simulink model "acc_decision_matlab_function"  (R2024b)
settings: Solver=FixedStepDiscrete  StartTime=0.0  StopTime=0.2  FixedStep=0.05  RelTol=1e-3
settings Model: Creator=aiden  LastModifiedBy=aiden
settings DataIOCC: ExternalInput=command_input, ego_speed_kmh, has_target, current_distance, reset_signal  LoadExternalInput=on

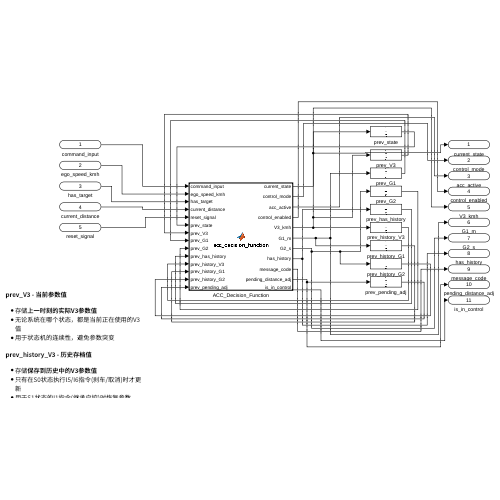
[thumbnail: Simulink's stored preview of the top-level diagram]
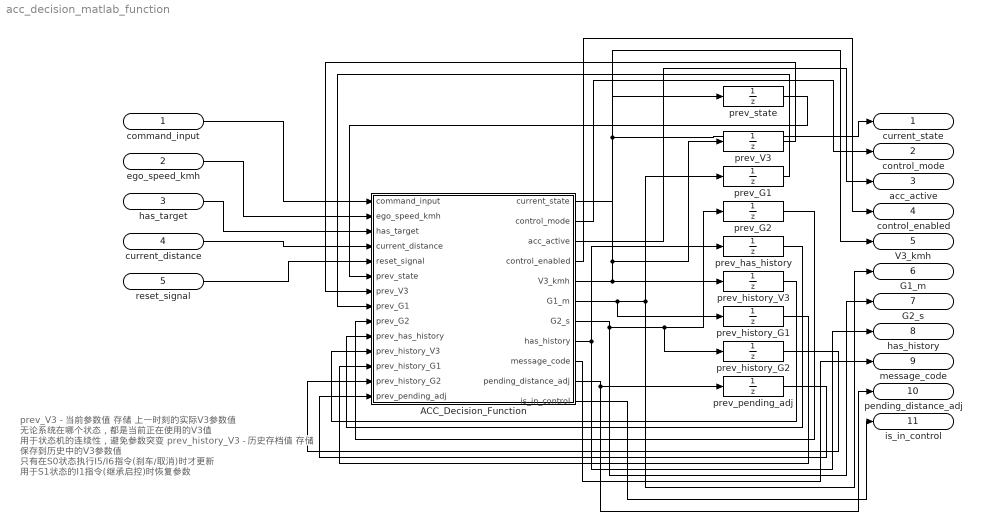
== system acc_decision_matlab_function ==
  note: prev_V3 - 当前参数值
      | 存储 上一时刻的实际V3参数值
      | 无论系统在哪个状态，都是当前正在使用的V3值
      | 用于状态机的连续性，避免参数突变
      | prev_history_V3 - 历史存档值
      | 存储 保存到历史中的V3参数值
      | 只有在S0状态执行I5/I6指令(刹车/取消)时才更新
      | 用于S1状态的I1指令(继承启控)时恢复参数
  command_input : Inport
  ego_speed_kmh : Inport  Port=2
  has_target : Inport  Port=3
  current_distance : Inport  Port=4
  reset_signal : Inport  Port=5
  ACC_Decision_Function : MATLAB Function  TreatAsAtomicUnit=on
  prev_G1 : UnitDelay  InitialCondition=15.0  SampleTime=-1  HasFrameUpgradeWarning=on
  prev_G2 : UnitDelay  InitialCondition=2.0  SampleTime=-1  HasFrameUpgradeWarning=on
  prev_V3 : UnitDelay  InitialCondition=50.0  SampleTime=-1  HasFrameUpgradeWarning=on
  prev_has_history : UnitDelay  InitialCondition=false  SampleTime=-1  HasFrameUpgradeWarning=on
  prev_history_G1 : UnitDelay  InitialCondition=15.0  SampleTime=-1  HasFrameUpgradeWarning=on
  prev_history_G2 : UnitDelay  InitialCondition=2.0  SampleTime=-1  HasFrameUpgradeWarning=on
  prev_history_V3 : UnitDelay  InitialCondition=50.0  SampleTime=-1  HasFrameUpgradeWarning=on
  prev_pending_adj : UnitDelay  SampleTime=-1  HasFrameUpgradeWarning=on
  prev_state : UnitDelay  InitialCondition=2  SampleTime=-1  HasFrameUpgradeWarning=on
  current_state : Outport
  control_mode : Outport  Port=2
  acc_active : Outport  Port=3
  control_enabled : Outport  Port=4
  V3_kmh : Outport  Port=5
  G1_m : Outport  Port=6
  G2_s : Outport  Port=7
  has_history : Outport  Port=8
  message_code : Outport  Port=9
  pending_distance_adj : Outport  Port=10
  is_in_control : Outport  Port=11
  wires:
  command_input/1 -> ACC_Decision_Function/1(command_input)
  ACC_Decision_Function/1(current_state) -> current_state/1, prev_state/1
  ego_speed_kmh/1 -> ACC_Decision_Function/2(ego_speed_kmh)
  has_target/1 -> ACC_Decision_Function/3(has_target)
  current_distance/1 -> ACC_Decision_Function/4(current_distance)
  reset_signal/1 -> ACC_Decision_Function/5(reset_signal)
  prev_state/1 -> ACC_Decision_Function/6(prev_state)
  prev_V3/1 -> ACC_Decision_Function/7(prev_V3)
  prev_G1/1 -> ACC_Decision_Function/8(prev_G1)
  prev_G2/1 -> ACC_Decision_Function/9(prev_G2)
  prev_has_history/1 -> ACC_Decision_Function/10(prev_has_history)
  prev_history_V3/1 -> ACC_Decision_Function/11(prev_history_V3)
  prev_history_G1/1 -> ACC_Decision_Function/12(prev_history_G1)
  prev_history_G2/1 -> ACC_Decision_Function/13(prev_history_G2)
  prev_pending_adj/1 -> ACC_Decision_Function/14(prev_pending_adj)
  ACC_Decision_Function/2(control_mode) -> control_mode/1
  ACC_Decision_Function/3(acc_active) -> acc_active/1
  ACC_Decision_Function/4(control_enabled) -> control_enabled/1
  ACC_Decision_Function/5(V3_kmh) -> prev_history_V3/1, prev_V3/1, V3_kmh/1
  ACC_Decision_Function/6(G1_m) -> prev_history_G1/1, G1_m/1, prev_G1/1
  ACC_Decision_Function/7(G2_s) -> prev_history_G2/1, prev_G2/1, G2_s/1
  ACC_Decision_Function/8(has_history) -> has_history/1, prev_has_history/1
  ACC_Decision_Function/9(message_code) -> message_code/1
  ACC_Decision_Function/10(pending_distance_adj) -> prev_pending_adj/1, pending_distance_adj/1
  ACC_Decision_Function/11(is_in_control) -> is_in_control/1

== matlab function acc_decision_matlab_function/ACC_Decision_Function ==
  data: command_input input; current_state output; ego_speed_kmh input; has_target input; current_distance input; reset_signal input; prev_state input; prev_V3 input; prev_G1 input; prev_G2 input; prev_has_history input; prev_history_V3 input; prev_history_G1 input; prev_history_G2 input; prev_pending_adj input; control_mode output; acc_active output; control_enabled output; V3_kmh output; G1_m output; G2_s output; has_history output; message_code output; pending_distance_adj output; is_in_control output
function [current_state, control_mode, acc_active, control_enabled, V3_kmh, G1_m, G2_s, has_history, message_code, pending_distance_adj, is_in_control] = acc_decision_function(command_input, ego_speed_kmh, has_target, current_distance, reset_signal, prev_state, prev_V3, prev_G1, prev_G2, prev_has_history, prev_history_V3, prev_history_G1, prev_history_G2, prev_pending_adj)
%% ACC自适应巡航决策函数
%% 基于decision.md实现的完整状态机逻辑

%% 常量定义
V1_KMH = 30.0;        %% 适速/低速界限
V2_KMH = 30.0;        %% 降速下限参考
SPEED_STEP = 1.0;     %% 速度调整步长
DISTANCE_STEP = 1.0;  %% 距离调整步长

%% 初始化输出（使用上一时刻值）
current_state = prev_state;
control_mode = 0;
V3_kmh = prev_V3;
G1_m = prev_G1;
G2_s = prev_G2;
has_history = prev_has_history;
history_V3_kmh = prev_history_V3;
history_G1_m = prev_history_G1;
history_G2_s = prev_history_G2;
pending_adj = prev_pending_adj;
message_code = 0;
pending_distance_adj = pending_adj;

%% 处理重置信号（最高优先级）
if reset_signal
    current_state = 3;
    V3_kmh = 50.0;
    G1_m = 15.0;
    G2_s = 2.0;
    has_history = false;
    history_V3_kmh = 50.0;
    history_G1_m = 15.0;
    history_G2_s = 2.0;
    pending_adj = 0;
    control_mode = 0;
    message_code = 0;
    acc_active = false;
    control_enabled = false;
    is_in_control = false;
    pending_distance_adj = 0;
    return;
end

%% 参数边界验证
if V3_kmh <= 0, V3_kmh = 50.0; end
if G1_m <= 0, G1_m = 15.0; end

%% 处理驾驶指令
if command_input >= 0 && command_input <= 6
    switch current_state
        case 0  %% S0_IN_CONTROL
            switch command_input
                case 0
                    control_mode = 1;
                    V3_kmh = max(V2_KMH+1, V3_kmh - SPEED_STEP);
                    message_code = 101;
                case 1
                    control_mode = 2;
                    V3_kmh = min(120, V3_kmh + SPEED_STEP);
                    message_code = 102;
                case 2
                    control_mode = 3;
                    G1_m = max(5, G1_m - DISTANCE_STEP);
                    message_code = 103;
                case 3
                    control_mode = 4;
                    G1_m = min(50, G1_m + DISTANCE_STEP);
                    message_code = 104;
                case 4
                    control_mode = 7;
                    message_code = 107;
                case {5, 6}
                    control_mode = 8;
                    has_history = true;
                    history_V3_kmh = V3_kmh;
                    history_G1_m = G1_m;
                    history_G2_s = G2_s;
                    current_state = 1;
                    message_code = 108 + (command_input - 5);
            end
        case 1  %% S1_ADAPTIVE_HISTORY_STANDBY
            switch command_input
                case 0
                    control_mode = 5;
                    current_state = 0;
                    message_code = 205;
                case 1
                    control_mode = 6;
                    if has_history
                        V3_kmh = history_V3_kmh;
                        G1_m = history_G1_m;
                        G2_s = history_G2_s;
                        if pending_adj ~= 0
                            G1_m = max(5.0, min(50.0, G1_m + pending_adj));
                            pending_adj = 0;
                        end
                    end
                    current_state = 0;
                    message_code = 206;
                otherwise
                    control_mode = 8;
                    message_code = 200 + command_input;
            end
        case 2  %% S2_ADAPTIVE_NO_HISTORY_STANDBY
            switch command_input
                case 0
                    control_mode = 5;
                    current_state = 0;
                    message_code = 305;
                otherwise
                    control_mode = 8;
                    message_code = 300 + command_input;
            end
        case 3  %% S3_LOW_SPEED
            if ego_speed_kmh < V1_KMH
                control_mode = 8;
                message_code = 400 + command_input;
            end
    end
end

%% 速度相关的自动状态转移
if ego_speed_kmh < V1_KMH && (current_state == 1 || current_state == 2)
    current_state = 3;
    message_code = 910 + current_state;
elseif ego_speed_kmh >= V1_KMH && current_state == 3
    if has_history
        current_state = 1;
        message_code = 931;
    else
        current_state = 2;
        message_code = 932;
    end
end

%% 设置状态相关的输出标志
switch current_state
    case 0
        acc_active = true;
        control_enabled = true;
        is_in_control = true;
    case {1, 2, 3}
        acc_active = false;
        control_enabled = false;
        is_in_control = false;
end

pending_distance_adj = pending_adj;

%% 处理未使用的输入以避免警告
if has_target || current_distance > 0
    %% 输入已使用
end
end
